simulink model "forwarddyn_1dof_2020a"  (R2020a)
settings: Solver=VariableStepAuto  StartTime=0.0  StopTime=10.0  FixedStep=0.0001  RelTol=1e-3  EnableMultiTasking=on
settings Model: Creator=shb  LastModifiedBy=CG88UN
settings DataIOCC: LimitDataPoints=on  SaveFormat=Array  ReturnWorkspaceOutputs=off
settings OptimizationCC: LifeSpan=inf
settings DebuggingCC: SFUnexpectedBacktrackingDiag=warning  SFNoUnconditionalDefaultTransitionDiag=warning  SFExecutionAtInitializationDiag=none  ArithmeticOperatorsInVariantConditions=warning
settings HardwareCC: ProdBitPerPointer=32  ProdBitPerSizeT=32  ProdBitPerPtrDiffT=32  ProdLargestAtomicFloat=None  ProdIntDivRoundTo=Undefined  ProdEndianess=Unspecified  ProdWordSize=32  ProdHWDeviceType=32-bit Generic
settings ModelReferenceCC: PropagateSignalLabelsOutOfModel=off
settings SFSimCC: SimUseLocalCustomCode=off  CustomCodeUndefinedFunction=UseInterfaceOnly
settings RTWCC: RTWUseLocalCustomCode=off
settings CodeAppCC: StateflowObjectComments=on
settings GRTTargetCC: TargetLangStandard=C89/C90 (ANSI)
settings ConfigComp: CovMetricSettings=dw  CovSaveCumulativeToWorkspaceVar=on  CovSaveSingleToWorkspaceVar=on  CovExternalEMLEnable=off

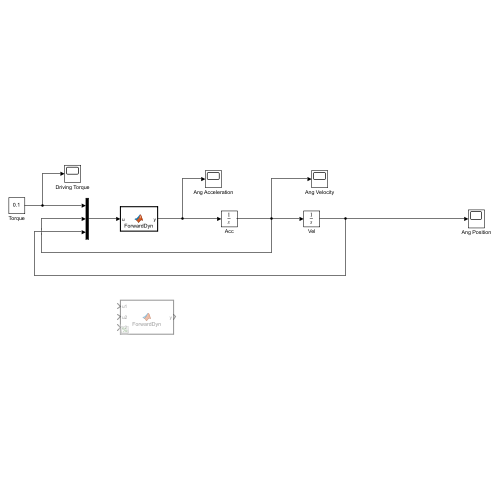
[thumbnail: Simulink's stored preview of the top-level diagram]
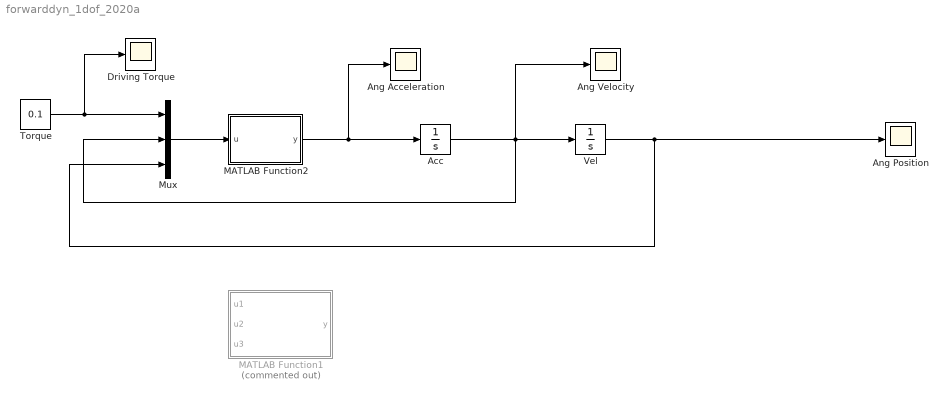
== system forwarddyn_1dof_2020a ==
  Acc : Integrator
  Ang Acceleration : Scope
  Ang Position : Scope
  Ang Velocity : Scope
  Driving Torque : Scope
  MATLAB Function1 : MATLAB Function  Commented=on  TreatAsAtomicUnit=on
  MATLAB Function2 : MATLAB Function  TreatAsAtomicUnit=on
  Mux : Mux  Inputs=3
  Torque : Constant  Value=0.1
  Vel : Integrator
  wires:
  Torque/1 -> Driving Torque/1, Mux/1
  Mux/1 -> MATLAB Function2/1(u)
  MATLAB Function2/1(y) -> Ang Acceleration/1, Acc/1
  Acc/1 -> Ang Velocity/1, Mux/2, Vel/1
  Vel/1 -> Mux/3, Ang Position/1

== matlab function forwarddyn_1dof_2020a/MATLAB Function2 ==
  data: u input; y output
function y = ForwardDyn(u)

%%   motor torques
tau_1 = u(1);

%% joint velocity and displacement
dtheta_1 = u(2); theta_1 = u(3); 

%%  %%%%%%%%%%%%%%%%%%%%%%%  motion profiles
% %=======================  joint 1
% A1 = 0.3; % magnitude
% f1 = 5; % frequency
% 
% %=======================  joint 2
% A2 = 0.5; % magnitude
% f2 = 2; % frequency

g = 9.801; % gravity constant

%% %%%%%%%%%%%%%%%%%%%%%%%%%%%%  link properties
%======================================  link 1
L1 = 0.5; % length [m]
c1 = L1/2; % mass center
m1 = 4.6; % mass [kg]
I1 = 1/12*m1*L1^2; % moment of inertia

%% %%%%%%%%%%%%%%%%%% dynamic simulation

    %%%%%%%%%%%%%%%%%%%%%%%%%%%  coefficients of dynamic equation
    H = m1*c1^2 + I1;
    G1 = m1*c1*g*cos(theta_1); 
    
    
%     %%%%%%%%%%%%%%%%%%%%%%%%%%%%%%%%%%%%%  actuator torques
%     tau_1 = H11*ddtheta_1 + H12*ddtheta_2 - h*(dtheta_2)^2 ...
%         -2*h*dtheta_1*dtheta_2 + G1;
%     tau_2 = H22*ddtheta_2 + H12*ddtheta_1 + h*(dtheta_1)^2 + G2;
    
    J = H; 
    torque = tau_1 + G1;
    
    y = J\torque;

== matlab function forwarddyn_1dof_2020a/MATLAB Function1 ==
  data: u1 input; y output; u2 input; u3 input
function y = ForwardDyn(u1,u2,u3)

%%   motor torques
tau_1 = u1;

%% joint velocity and displacement
dtheta_1 = u2; theta_1 = u2; 

%%  %%%%%%%%%%%%%%%%%%%%%%%  motion profiles
% %=======================  joint 1
% A1 = 0.3; % magnitude
% f1 = 5; % frequency
% 
% %=======================  joint 2
% A2 = 0.5; % magnitude
% f2 = 2; % frequency

g = 9.801; % gravity constant

%% %%%%%%%%%%%%%%%%%%%%%%%%%%%%  link properties
%======================================  link 1
L1 = 0.5; % length [m]
c1 = L1/2; % mass center
m1 = 4.6; % mass [kg]
I1 = 1/12*m1*L1^2; % moment of inertia

%% %%%%%%%%%%%%%%%%%% dynamic simulation

    %%%%%%%%%%%%%%%%%%%%%%%%%%%  coefficients of dynamic equation
    H = m1*c1^2 + I1;
    G1 = m1*c1*g*cos(theta_1); 
    
    
%     %%%%%%%%%%%%%%%%%%%%%%%%%%%%%%%%%%%%%  actuator torques
%     tau_1 = H11*ddtheta_1 + H12*ddtheta_2 - h*(dtheta_2)^2 ...
%         -2*h*dtheta_1*dtheta_2 + G1;
%     tau_2 = H22*ddtheta_2 + H12*ddtheta_1 + h*(dtheta_1)^2 + G2;
    
    J = H; 
    torque = tau_1 + G1;
    
    y = J\torque;
